simulink model "ramp_step"  (R2021a)
settings: Solver=VariableStepAuto  StartTime=0.0  StopTime=20  RelTol=1e-3
libraries: simulink x2
settings Model: Creator=Beshary  LastModifiedBy=Beshary

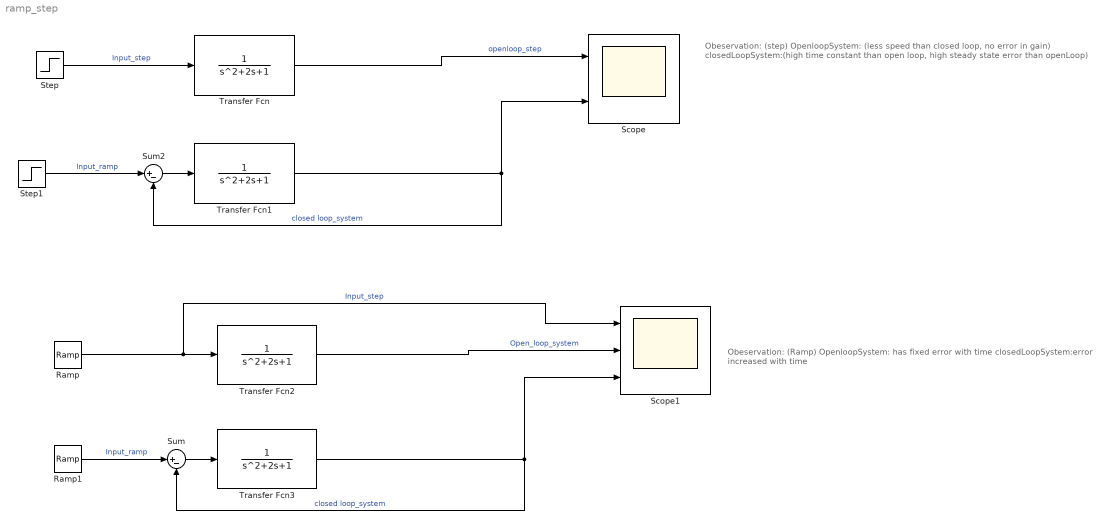
== system ramp_step ==
  note: Obeservation: (Ramp)
      | OpenloopSystem: has fixed error with time
      | closedLoopSystem:error increased with time
  note: Obeservation: (step)
      | OpenloopSystem: (less speed than closed loop, no error in gain)
      | closedLoopSystem:(high time constant than open loop, high steady state error than openLoop)
  Ramp : simulink/Sources/Ramp  slope=1  start=0  InitialOutput=0
  Ramp1 : simulink/Sources/Ramp  slope=1  start=0  InitialOutput=0
  Scope : Scope  NumInputPorts=2
  Scope1 : Scope  NumInputPorts=3
  Step : Step  SampleTime=0
  Step1 : Step  SampleTime=0
  Sum : Sum  Inputs=|+-
  Sum2 : Sum  Inputs=|+-
  Transfer Fcn{,1..3} (4 alike) : TransferFcn
  wires:
  Step/1 -> Transfer Fcn/1  "Input_step"
  Transfer Fcn/1 -> Scope/1  "openloop_step"
  Transfer Fcn3/1 -> Sum/2, Scope1/3  "closed loop_system"
  Transfer Fcn2/1 -> Scope1/2  "Open_loop_system"
  Ramp1/1 -> Sum/1  "Input_ramp"
  Ramp/1 -> Scope1/1, Transfer Fcn2/1  "Input_step"
  Sum/1 -> Transfer Fcn3/1
  Sum2/1 -> Transfer Fcn1/1
  Step1/1 -> Sum2/1  "Input_ramp"
  Transfer Fcn1/1 -> Sum2/2, Scope/2  "closed loop_system"
